simulink model "test_NO_OBSERVER_random"  (R2020a)
settings: Solver=ode15s  StartTime=0.0  StopTime=15  FixedStep=1/fs  MaxStep=1/(fs)  RelTol=1e-6
undefined symbols (not defined in the file): A, B, ba, Cc, D, den_anti, den_mems, f0, fs, g, K_motor_virtual, ksi, ksia, L, n_adc, NSD_mems, num_anti, num_mems, R, R_control, rms_rand, sens_mems, v0, Vcc, Vmax_ADC, Vmin_ADC, x0
libraries: simulink x2, dspstat3 x1, simulink_extras x1
settings Model: Creator=Noxi-PC  LastModifiedBy=Noxi-PC
settings SolverCC: ZeroCrossAlgorithm=Adaptive
settings DebuggingCC: IgnoredZcDiagnostic=none

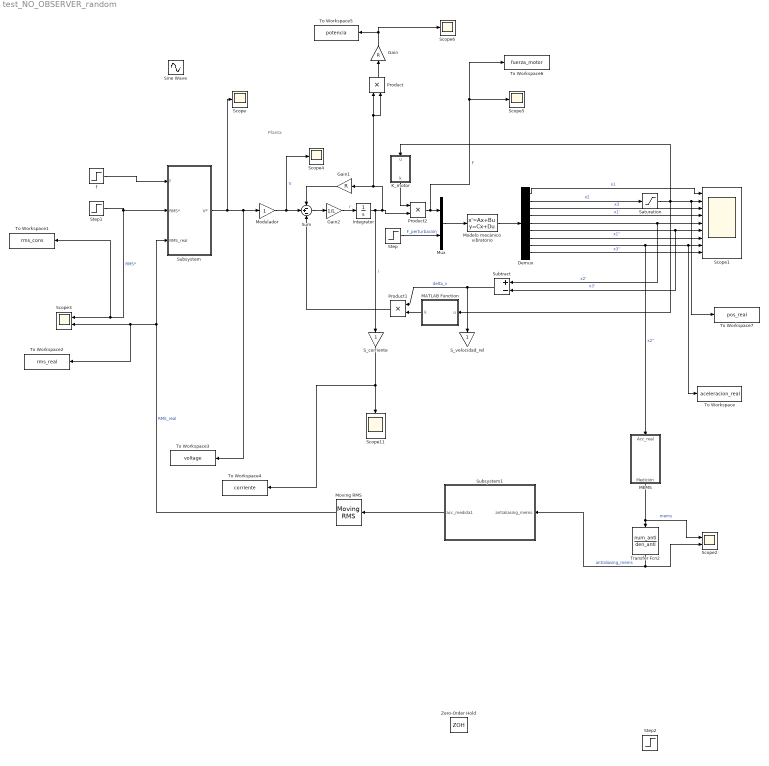
== system test_NO_OBSERVER_random ==
  note: Planta
  Demux : Demux  Outputs=9
  Gain : Gain  Gain=R
  Gain1 : Gain  Gain=R
  Gain2 : Gain  Gain=1/L
  Integrator : Integrator
  K_motor : MATLAB Function  TreatAsAtomicUnit=on
  MATLAB Function : MATLAB Function  TreatAsAtomicUnit=on
  MEMS : Subsystem
  Modelo mecánico vibratorio : StateSpace  A=A  B=B  C=Cc  D=D  InitialCondition=[x0,v0]
  Modulador : Gain
  Moving RMS : dspstat3/Moving RMS  Method=Sliding window  ForgettingFactorPort=off  SpecifyWindowLength=on  WindowLength=Ventana  ForgettingFactor=0.99  SimulateUsing=Interpreted execution
      settings: SourceProductBaseCode=DS
  Mux : Mux  Inputs=2
  Product : Product
  Product1 : Product
  Product2 : Product
  S_corriente : Gain
  S_velocidad_rel : Gain
  Saturation : Saturate  UpperLimit=12.7e-3  LowerLimit=-12.7e-3
  Scope{,4..6,11} (5 alike) : Scope
  Scope1 : Scope  NumInputPorts=9
  Scope2 : Scope  NumInputPorts=2
  Scope3 : Scope  NumInputPorts=2
  Sine Wave : Sin  Amplitude=5  Frequency=2*pi*f0  SampleTime=0
  Step : Step  Time=3  After=0  SampleTime=0
  Step1 : Step  Time=0  After=rms_rand  SampleTime=0
  Step2 : Step  SampleTime=0
  Subsystem : Subsystem
  Subsystem1 : Subsystem
  Subtract : Sum  Inputs=+-
  Sum : Sum  Inputs=-+-
  To Workspace : ToWorkspace  VariableName=aceleracion_real  SaveFormat=Structure With Time  SampleTime=-1
  To Workspace1 : ToWorkspace  VariableName=rms_cons  SaveFormat=Structure With Time  SampleTime=-1
  To Workspace2 : ToWorkspace  VariableName=rms_real  SaveFormat=Structure With Time  SampleTime=-1
  To Workspace3 : ToWorkspace  VariableName=voltage  SaveFormat=Structure With Time  SampleTime=-1
  To Workspace4 : ToWorkspace  VariableName=corriente  SaveFormat=Structure With Time  SampleTime=-1
  To Workspace5 : ToWorkspace  VariableName=potencia  SaveFormat=Structure With Time  SampleTime=-1
  To Workspace6 : ToWorkspace  VariableName=fuerza_motor  SaveFormat=Structure With Time  SampleTime=-1
  To Workspace7 : ToWorkspace  VariableName=pos_real  SaveFormat=Structure With Time  SampleTime=-1
  Transfer Fcn2 : TransferFcn  Numerator=num_anti  Denominator=den_anti
  Zero-Order Hold : ZeroOrderHold  SampleTime=1/fs
  f : Step  Time=0  After=2000  SampleTime=0
  wires:
  Modelo mecánico vibratorio/1 -> Demux/1
  Demux/1 -> Scope1/1  "x1"
  Demux/2 -> Saturation/1  "x2"
  Demux/3 -> Scope1/3  "x3"
  Demux/4 -> Scope1/4  "x1'"
  Demux/5 -> Scope1/5, Subtract/1  "x2'"
  Demux/6 -> Scope1/6, Subtract/2  "x3'"
  Demux/7 -> Scope1/7  "x1''"
  Demux/8 -> MEMS/1(Acc_real), To Workspace/1, Scope1/8  "x2''"
  Demux/9 -> Scope1/9  "x3''"
  Mux/1 -> Modelo mecánico vibratorio/1
  Sum/1 -> Gain2/1
  Integrator/1 -> S_corriente/1, Product2/2, Gain1/1, Product/2, Product/1  "i"
  Gain1/1 -> Sum/1
  Gain2/1 -> Integrator/1  "i'"
  Step/1 -> Mux/2  "F_perturbación"
  Product1/1 -> Sum/3
  Subtract/1 -> Product1/1, S_velocidad_rel/1  "delta_v"
  Modulador/1 -> Scope4/1, Sum/2  "V"
  Saturation/1 -> K_motor/1(u), MATLAB Function/1(u), To Workspace7/1, Scope1/2
  Product2/1 -> To Workspace6/1, Scope5/1, Mux/1  "F"
  K_motor/1(k) -> Product2/1
  MATLAB Function/1(k) -> Product1/2
  f/1 -> Subsystem/1(f)
  Step1/1 -> Subsystem/2(RMS*), To Workspace1/1, Scope3/1  "RMS*"
  Subsystem/1(V*') -> Scope/1, To Workspace3/1, Modulador/1
  MEMS/1(Medición) -> Scope2/1, Transfer Fcn2/1  "mems"
  Moving RMS/1 -> Subsystem/3(RMS_real), To Workspace2/1, Scope3/2  "RMS_real"
  Transfer Fcn2/1 -> Scope2/2, Subsystem1/1(antialiasing_mems)  "antialiasing_mems"
  S_corriente/1 -> To Workspace4/1, Scope11/1
  Product/1 -> Gain/1
  Gain/1 -> To Workspace5/1, Scope6/1
  Subsystem1/1(acc_medida1) -> Moving RMS/1

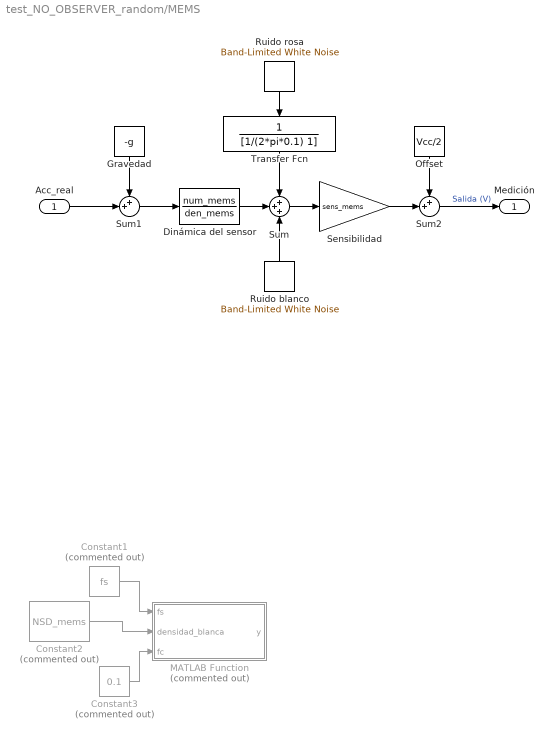
== system test_NO_OBSERVER_random/MEMS ==
  Acc_real : Inport
  Constant1 : Constant  Commented=on  Value=fs
  Constant2 : Constant  Commented=on  Value=NSD_mems
  Constant3 : Constant  Commented=on  Value=0.1
  Dinámica del sensor : TransferFcn  Numerator=num_mems  Denominator=den_mems
  Gravedad : Constant  Value=-g
  MATLAB Function : MATLAB Function  Commented=on  TreatAsAtomicUnit=on
  Offset : Constant  Value=Vcc/2
  Ruido blanco : simulink/Sources/Band-Limited White Noise  Cov=PSD_mems  Ts=3/50*1/fs  seed=[2674]
  Ruido rosa : simulink/Sources/Band-Limited White Noise  Cov=PSD_mems  Ts=3/50*1/fs  seed=[26744]
  Sensibilidad : Gain  Gain=sens_mems
  Sum : Sum  Inputs=+++
  Sum1 : Sum  Inputs=++|
  Sum2 : Sum  Inputs=++|
  Transfer Fcn : TransferFcn  Denominator=[1/(2*pi*0.1) 1]
  Medición : Outport
  wires:
  Sum1/1 -> Dinámica del sensor/1
  Acc_real/1 -> Sum1/2
  Sum/1 -> Sensibilidad/1
  Sensibilidad/1 -> Sum2/2
  Sum2/1 -> Medición/1  "Salida (V)"
  Gravedad/1 -> Sum1/1
  Offset/1 -> Sum2/1
  Constant1/1 -> MATLAB Function/1(fs)
  Constant2/1 -> MATLAB Function/2(densidad_blanca)
  Constant3/1 -> MATLAB Function/3(fc)
  Ruido blanco/1 -> Sum/3
  Ruido rosa/1 -> Transfer Fcn/1
  Dinámica del sensor/1 -> Sum/2
  Transfer Fcn/1 -> Sum/1

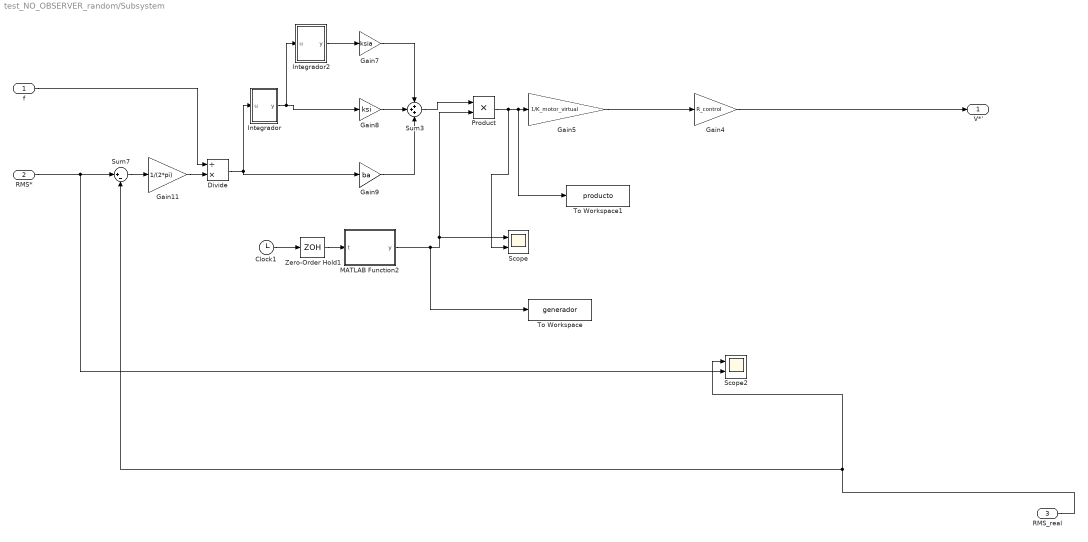
== system test_NO_OBSERVER_random/Subsystem ==
  f : Inport
  RMS* : Inport  Port=2
  RMS_real : Inport  Port=3
  Clock1 : Clock
  Divide : Product  Inputs=/*
  Gain11 : Gain  Gain=1/(2*pi)
  Gain4 : Gain  Gain=R_control
  Gain5 : Gain  Gain=1/K_motor_virtual
  Gain7 : Gain  Gain=ksia
  Gain8 : Gain  Gain=ksi
  Gain9 : Gain  Gain=ba
  Integrador : Subsystem
  Integrador2 : Subsystem
  MATLAB Function2 : MATLAB Function  TreatAsAtomicUnit=on
  Product : Product
  Scope : Scope  NumInputPorts=2
  Scope2 : Scope  NumInputPorts=2
  Sum3 : Sum  Inputs=+++
  Sum7 : Sum  Inputs=|+-
  To Workspace : ToWorkspace  VariableName=generador  SaveFormat=Structure With Time  SampleTime=-1
  To Workspace1 : ToWorkspace  VariableName=producto  SaveFormat=Structure With Time  SampleTime=-1
  Zero-Order Hold1 : ZeroOrderHold  SampleTime=1/fs
  V*' : Outport
  wires:
  Integrador2/1(y) -> Gain7/1
  Integrador/1(y) -> Gain8/1, Integrador2/1(u)
  RMS_real/1 -> Scope2/1, Sum7/2
  RMS*/1 -> Scope2/2, Sum7/1
  Gain8/1 -> Sum3/2
  Gain9/1 -> Sum3/3
  Sum7/1 -> Gain11/1
  f/1 -> Divide/1
  Sum3/1 -> Product/1
  Product/1 -> Scope/2, To Workspace1/1, Gain5/1
  Gain5/1 -> Gain4/1
  Gain11/1 -> Divide/2
  Gain7/1 -> Sum3/1
  Divide/1 -> Integrador/1(u), Gain9/1
  MATLAB Function2/1(y) -> To Workspace/1, Product/2, Scope/1
  Clock1/1 -> Zero-Order Hold1/1
  Zero-Order Hold1/1 -> MATLAB Function2/1(t)
  Gain4/1 -> V*'/1

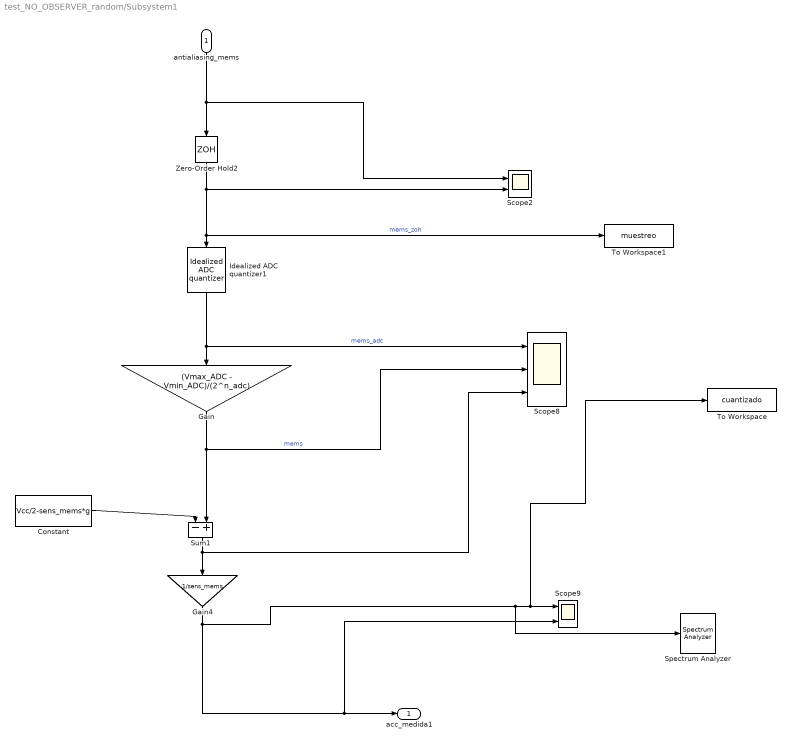
== system test_NO_OBSERVER_random/Subsystem1 ==
  antialiasing_mems : Inport
  Constant : Constant  Value=Vcc/2-sens_mems*g
  Gain : Gain  Gain=(Vmax_ADC - Vmin_ADC)/(2^n_adc)
  Gain4 : Gain  Gain=1/sens_mems
  Idealized ADC quantizer1 : simulink_extras/Additional Discrete/Idealized ADC quantizer  NumberOfConverterBits=n_adc  Vmin=Vmin_ADC  Vmax=Vmax_ADC  OutputDataType=uint16  OutputNegativeValues=off
  Scope2 : Scope  NumInputPorts=2
  Scope8 : Scope  NumInputPorts=3
  Scope9 : Scope  NumInputPorts=2
  Spectrum Analyzer : SpectrumAnalyzer
  Sum1 : Sum  Inputs=-+
  To Workspace : ToWorkspace  VariableName=cuantizado  SaveFormat=Structure With Time  SampleTime=1/fs
  To Workspace1 : ToWorkspace  VariableName=muestreo  SaveFormat=Structure With Time  SampleTime=1/fs
  Zero-Order Hold2 : ZeroOrderHold  SampleTime=1/(fs)
  acc_medida1 : Outport
  wires:
  Gain/1 -> Scope8/2, Sum1/2  "mems"
  Idealized ADC quantizer1/1 -> Gain/1, Scope8/1  "mems_adc"
  Sum1/1 -> Scope8/3, Gain4/1
  antialiasing_mems/1 -> Scope2/1, Zero-Order Hold2/1
  Zero-Order Hold2/1 -> To Workspace1/1, Idealized ADC quantizer1/1, Scope2/2  "mems_zoh"
  Gain4/1 -> Scope9/2, acc_medida1/1, To Workspace/1, Scope9/1, Spectrum Analyzer/1
  Constant/1 -> Sum1/1

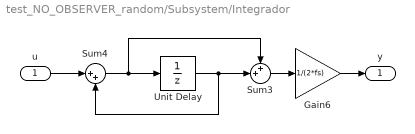
== system test_NO_OBSERVER_random/Subsystem/Integrador ==
  u : Inport
  Gain6 : Gain  Gain=1/(2*fs)
  Sum3 : Sum  Inputs=++|
  Sum4 : Sum  Inputs=|++
  Unit Delay : UnitDelay  SampleTime=1/fs  HasFrameUpgradeWarning=on
  y : Outport
  wires:
  Sum3/1 -> Gain6/1
  Sum4/1 -> Sum3/1, Unit Delay/1
  Unit Delay/1 -> Sum3/2, Sum4/2
  Gain6/1 -> y/1
  u/1 -> Sum4/1

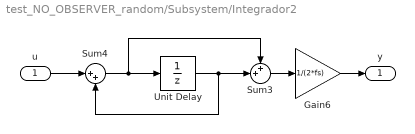
== system test_NO_OBSERVER_random/Subsystem/Integrador2 ==
  u : Inport
  Gain6 : Gain  Gain=1/(2*fs)
  Sum3 : Sum  Inputs=++|
  Sum4 : Sum  Inputs=|++
  Unit Delay : UnitDelay  SampleTime=1/fs  HasFrameUpgradeWarning=on
  y : Outport
  wires:
  Sum3/1 -> Gain6/1
  Sum4/1 -> Sum3/1, Unit Delay/1
  Unit Delay/1 -> Sum3/2, Sum4/2
  Gain6/1 -> y/1
  u/1 -> Sum4/1

== matlab function test_NO_OBSERVER_random/MATLAB Function ==
  data: u input; k output
function k= fcn(u)
coefs = [1883883250149.81,121220914.941173,-604988778.285297,-369001.905871325,-43371.4523559472,-47.4444922489166,51.4222931299995];

k = coefs(1)*u^6+coefs(2)*u^5+coefs(3)*u^4+coefs(4)*u^3+coefs(5)*u^2+coefs(6)*u^1+coefs(7);

== matlab function test_NO_OBSERVER_random/MEMS/MATLAB Function ==
  data: fs input; y output; densidad_blanca input; fc input
function y = ruido_sensor(fs, densidad_blanca, fc)

% Persistent state
persistent b a z

if isempty(b)
    [b, a] = butter(1, fc/(fs/2));
    z = 0;  % Estado inicial del filtro
end

% Ruido blanco
ruido_blanco = densidad_blanca * randn * sqrt(fs);

% Ruido 1/f (drift)
[ruido_drift, z] = filter(b, a, randn, z);

% Señal total
y = ruido_blanco + ruido_drift;

== matlab function test_NO_OBSERVER_random/Subsystem/MATLAB Function2 ==
  data: y output; t input
function y = GeneradorPerfilPSD(t)
% Genera una señal aleatoria con un perfil PSD deseado
% Entrada: t (Simulink le pasa el tiempo automáticamente)
% Salida: y (valor de aceleración en ese instante)

persistent f_list A_list phi_list t0

% Definir perfil PSD solo una vez
if isempty(f_list)
    % Tramos del perfil (frecuencias en Hz)
    freqs = [20, 130, 800, 2000];                 % Bordes
    psd_vals = [0.01125, 0.05625, 0.05625, 0.015]; % [g²/Hz]

    % Parámetros del generador
    Ncomp = 100;  % Número total de componentes senoidales
    rng(5);       % Semilla fija para reproducibilidad

    % Generar frecuencias espaciadas entre 20 y 2000 Hz
    f_list = linspace(freqs(1), freqs(end), Ncomp);

    % Calcular PSD escalonada (por tramos planos)
    psd_interp = zeros(size(f_list));
    for i = 1:length(freqs)-1
        idx = (f_list >= freqs(i)) & (f_list < freqs(i+1));
        psd_interp(idx) = psd_vals(i);
    end
    psd_interp(end) = psd_vals(end);

    % Calcular amplitudes: A = sqrt(2 * PSD * df)
    df = mean(diff(f_list));
    A_list = sqrt(2 * psd_interp * df)*9.81;

    % Fases aleatorias
    phi_list = 2 * pi * rand(1, Ncomp);

    % Tiempo inicial
    t0 = t;
end

% Generar la señal
y = sum(A_list .* sin(2*pi*f_list*(t - t0) + phi_list));

== matlab function test_NO_OBSERVER_random/K_motor ==
  data: u input; k output
function k = fcn(u)
coefs = [1.88388325014986e-06,1.21220914940963e-07,-0.000604988778285308,-0.000369001905871298,-0.0433714523559467,-0.0474444922489168,51.4222931299995];

k = coefs(1)*u^6+coefs(2)*u^5+coefs(3)*u^4+coefs(4)*u^3+coefs(5)*u^2+coefs(6)*u^1+coefs(7);
